simulink model "TxSteering_RxMVDR_4x4_HDL_IQ"  (R2021b)
settings: Solver=FixedStepDiscrete  StartTime=0.0  StopTime=stoptime  RelTol=1e-3
PreLoadFcn:
  | model_init
InitFcn:
  | model_init
model workspace (MAT data in the model file):
  socvcb = containers.Map
  socvcb.serialization.keys = {}
  socvcb.serialization.values = {}
  socvcb.serialization.uniformity = 0
  socvcb.serialization.keyType = 'double'
  socvcb.serialization.valueType = 'any'
values from neighbouring files (symbols this model uses):
  fc = ConverterSampleRate/4    (= 491520000)    [model_init.m]
  FPGAClkRate = DataSampleRate/VectorSamplingFactor    (= 245760000)    [model_init.m]
  movavg_bitshift = nextpow2(sqrt(windowSize))    [model_init.m]
  mvdrPipelineDelay = covMatDelay+movAvgDelay+matrixDivDelay+normResponseDelay    [model_init.m]
  NCO_bits = 14    [model_init.m]
  numArrayElements = 4    [model_init.m]
  S2MM_frame_size = testSrc1.FrameLength*testSrc1.SamplesPerSymbol*3    [model_init.m]
  testSrc1 = struct()    [model_init.m]
  testSrc2 = struct()    [model_init.m]
  windowSize = 4096    [model_init.m]
undefined symbols (not defined in the file or in its folder): j, physconst
libraries: hdlsllib x19, simulink x12, dspsrcs4 x2, embsystolicmatrixops x1, embreciprocals x1, dsphdlsigops x1, commrfcorlib x1
(part 1 of 3)
Description:
  | MVDR RFSoC example for ZCU111
  | 
  | Copyright 2021 The MathWorks, Inc.
settings Model: DataTypeOverride=Off  Creator=mfornero  LastModifiedBy=tmealey
settings SolverCC: AlgebraicLoopSolver=TrustRegion
settings DataIOCC: SaveOutput=off  SaveTime=off  ReturnWorkspaceOutputs=off
settings OptimizationCC: BlockReduction=off  ConditionallyExecuteInputs=off  DefaultParameterBehavior=Inlined  LifeSpan=inf
settings DebuggingCC: AlgebraicLoopMsg=error  SingleTaskRateTransMsg=error  ParameterPrecisionLossMsg=none  PregeneratedLibrarySubsystemCodeDiagnostic=none  StrictBusMsg=ErrorOnBusTreatedAsVector  SFUnexpectedBacktrackingDiag=warning  SFNoUnconditionalDefaultTransitionDiag=warning  SFExecutionAtInitializationDiag=none  SFMachineParentedDataDiag=warning  ArithmeticOperatorsInVariantConditions=warning
settings HardwareCC: ProdBitPerPointer=32  ProdBitPerSizeT=32  ProdBitPerPtrDiffT=32  ProdLargestAtomicFloat=None  ProdIntDivRoundTo=Undefined  ProdEndianess=Unspecified  ProdWordSize=32  ProdHWDeviceType=ASIC/FPGA->ASIC/FPGA  ProdEqTarget=off
settings SFSimCC: SimUseLocalCustomCode=off  CustomCodeUndefinedFunction=UseInterfaceOnly
settings RTWCC: RTWUseLocalCustomCode=off
settings CodeAppCC: StateflowObjectComments=on
settings GRTTargetCC: TargetLangStandard=C89/C90 (ANSI)
settings ConfigComp: CovMetricSettings=dw  CovSaveCumulativeToWorkspaceVar=on  CovSaveSingleToWorkspaceVar=on  CovExternalEMLEnable=off

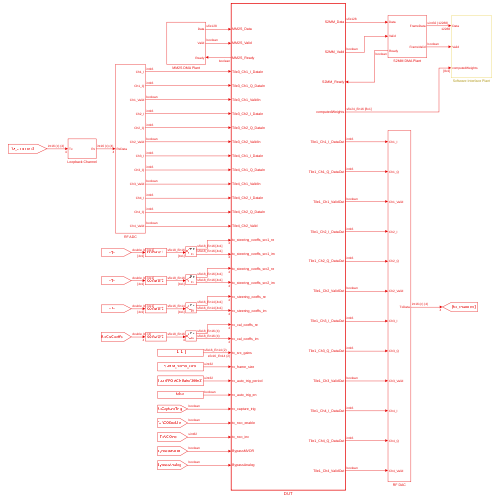
[thumbnail: Simulink's stored preview of the top-level diagram]
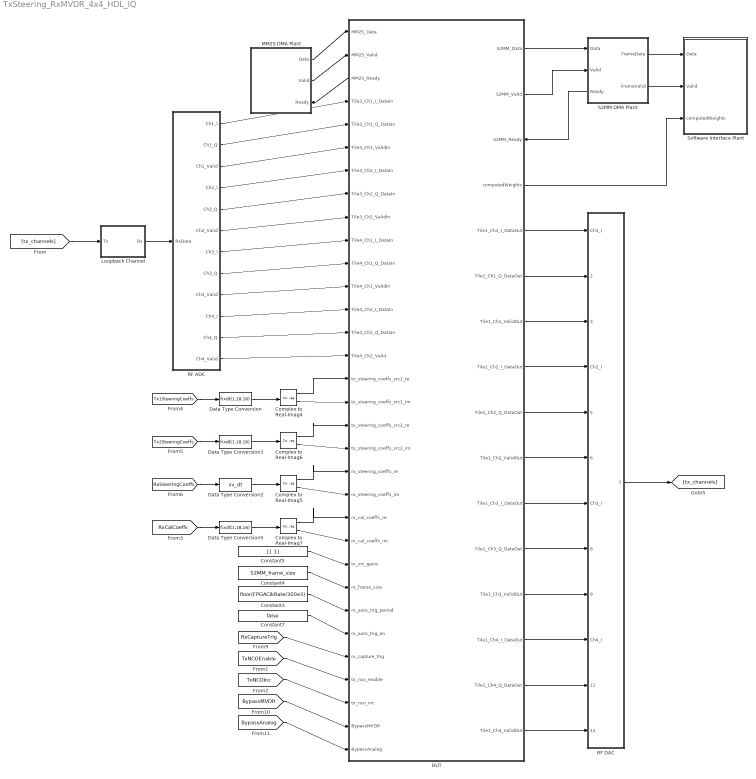
== system TxSteering_RxMVDR_4x4_HDL_IQ ==
  Complex to Real-Imag{4..7} (4 alike) : ComplexToRealImag
  Constant3 : Constant  Value=floor(FPGAClkRate/300e3)  OutDataTypeStr=uint32  SampleTime=-1
  Constant4 : Constant  Value=S2MM_frame_size  OutDataTypeStr=uint32  SampleTime=-1
  Constant5 : Constant  Value=[1 1]  OutDataTypeStr=tx_gain_dt  SampleTime=-1
  Constant7 : Constant  Value=false  SampleTime=-1
  DUT : Subsystem  TreatAsAtomicUnit=on
      settings: PortSchema="{\"entries\":[{\"content\":{\"sides\":[{\"content\":{\"connectorIds\":[\"In1\",\"In2\",\"Out16\",\"In3\",\"In4\",\"In5\",\"In6\",\"In7\",\"In8\",\"In9\",\"In10\",\"In11\",\"In12\",\"In13\",\"In14\",\"In15\",\"In16\",\"In17\",\"In18\",\"In19\",\"In20\",\"In21\",\"In22\",\"In23\",\"In24\",\"In25\",\"In26\",\"In27\",\"In28\",\"In29\",\"In30\",\"In31\"]},\"type\":\"ConnectorPlacement.EquallySpacedRectSide\",\"uuid\":\"5cbbc5c1-13a2-4dd5-b798-0d6aa5a3512c\"},{\"content\":{\"connectorIds\":[\"Out1\",\"Out2\",\"In32\",\"Out3\",\"Out4\",\"Out5\",\"Out6\",\"Out7\",\"Out8\",\"Out9\",\"Out10\",\"Out11\",\"Out12\",\"Out13\",\"Out14\",\"Out15\"],\"side\":\"RIGHT\"},\"type\":\"ConnectorPlacement.EquallySpacedRectSide\",\"uuid\":\"078c6bc6-159b-4e6a-9020-aaf50b1c87f6\"},{\"content\":{\"connectorIds\":[],\"side\":\"TOP\"},\"type\":\"ConnectorPlacement.EquallySpacedRectSide\",\"uuid\":\"5dec20bf-c028-4555-acb0-00d4e0bd1eb1\"},{\"content\":{\"connectorIds\":[],\"side\":\"HIDDEN\"},\"type\":\"ConnectorPlacement.EquallySpacedRectSide\",\"uuid\":\"f104c99f-3c00-46d1-a3ab-da9a095ae20c\"}]},\"type\":\"ConnectorPlacement.EquallySpacedConnector\",\"uuid\":\"99ff154b-6e8c-428f-8f67-53aff3cd9053\"}],\"packageUris\":[\"http://schema.mathworks.com/mf0/Connector/R2020b\"],\"version\":\"1.0\"}"
  Data Type Conversion : DataTypeConversion  OutDataTypeStr=fixdt(1,18,16)
  Data Type Conversion2 : DataTypeConversion  OutDataTypeStr=sv_dt
  Data Type Conversion3 : DataTypeConversion  OutDataTypeStr=fixdt(1,18,16)
  Data Type Conversion5 : DataTypeConversion  OutDataTypeStr=fixdt(1,18,16)
  Loopback Channel : Subsystem
  MM2S DMA Plant : Subsystem
      settings: PortSchema="{\"entries\":[{\"content\":{\"sides\":[{\"content\":{\"connectorIds\":[]},\"type\":\"ConnectorPlacement.EquallySpacedRectSide\",\"uuid\":\"6e5a1ec8-43bd-4e5c-bb67-adc7e52f765e\"},{\"content\":{\"connectorIds\":[\"Out1\",\"Out2\",\"In1\"],\"side\":\"RIGHT\"},\"type\":\"ConnectorPlacement.EquallySpacedRectSide\",\"uuid\":\"3e14b147-97a5-457d-828e-9dc648279d0e\"},{\"content\":{\"connectorIds\":[],\"side\":\"TOP\"},\"type\":\"ConnectorPlacement.EquallySpacedRectSide\",\"uuid\":\"b499ca48-b31e-4779-aede-04dca658d330\"},{\"content\":{\"connectorIds\":[],\"side\":\"HIDDEN\"},\"type\":\"ConnectorPlacement.EquallySpacedRectSide\",\"uuid\":\"e46e2562-9ab1-42db-980c-487b803af873\"}]},\"type\":\"ConnectorPlacement.EquallySpacedConnector\",\"uuid\":\"234057b8-4ead-4b5a-9893-76ff1204f271\"}],\"packageUris\":[\"http://schema.mathworks.com/mf0/Connector/R2020b\"],\"version\":\"1.0\"}"
  RF ADC : Subsystem
  RF DAC : Subsystem
  S2MM DMA Plant : Subsystem
      settings: PortSchema="{\"entries\":[{\"content\":{\"sides\":[{\"content\":{\"connectorIds\":[\"In1\",\"In2\",\"Out3\"]},\"type\":\"ConnectorPlacement.EquallySpacedRectSide\",\"uuid\":\"f5aebce5-d24c-432e-8d9d-6ae810fc0a64\"},{\"content\":{\"connectorIds\":[\"Out1\",\"Out2\"],\"side\":\"RIGHT\"},\"type\":\"ConnectorPlacement.EquallySpacedRectSide\",\"uuid\":\"87d7b61c-1b18-489c-87d0-263bc891b967\"},{\"content\":{\"connectorIds\":[],\"side\":\"TOP\"},\"type\":\"ConnectorPlacement.EquallySpacedRectSide\",\"uuid\":\"c0471b66-642d-47c1-93a8-85d0262e809a\"},{\"content\":{\"connectorIds\":[],\"side\":\"HIDDEN\"},\"type\":\"ConnectorPlacement.EquallySpacedRectSide\",\"uuid\":\"468d2625-6b9b-4b39-93eb-7f122a4e72a5\"}]},\"type\":\"ConnectorPlacement.EquallySpacedConnector\",\"uuid\":\"6af60fba-ab37-47d2-9d8a-dd48226214e6\"}],\"packageUris\":[\"http://schema.mathworks.com/mf0/Connector/R2020b\"],\"version\":\"1.0\"}"
  Software Interface Plant : Subsystem
  wires:
  Complex to Real-Imag4/2 -> DUT/16(tx_steering_coeffs_src1_im)
  [BypassAnalog] -> DUT/31(BypassAnalog)
  Complex to Real-Imag5/2 -> DUT/20(rx_steering_coeffs_im)
  Complex to Real-Imag6/2 -> DUT/18(tx_steering_coeffs_src2_im)
  Complex to Real-Imag6/1 -> DUT/17(tx_steering_coeffs_src2_re)
  Complex to Real-Imag5/1 -> DUT/19(rx_steering_coeffs_re)
  Data Type Conversion3/1 -> Complex to Real-Imag6/1
  Complex to Real-Imag4/1 -> DUT/15(tx_steering_coeffs_src1_re)
  Data Type Conversion2/1 -> Complex to Real-Imag5/1
  [Tx1SteeringCoeffs] -> Data Type Conversion/1
  Data Type Conversion/1 -> Complex to Real-Imag4/1
  Constant5/1 -> DUT/23(tx_src_gains)
  Constant7/1 -> DUT/26(rx_auto_trig_en)
  Constant3/1 -> DUT/25(rx_auto_trig_period)
  Constant4/1 -> DUT/24(rx_frame_size)
  [RxCaptureTrig] -> DUT/27(rx_capture_trig)
  Data Type Conversion5/1 -> Complex to Real-Imag7/1
  Complex to Real-Imag7/1 -> DUT/21(rx_cal_coeffs_re)
  Complex to Real-Imag7/2 -> DUT/22(rx_cal_coeffs_im)
  [RxCalCoeffs] -> Data Type Conversion5/1
  DUT/16(MM2S_Ready) -> MM2S DMA Plant/1(Ready)
  MM2S DMA Plant/2(Valid) -> DUT/2(MM2S_Valid)
  MM2S DMA Plant/1(Data) -> DUT/1(MM2S_Data)
  [BypassMVDR] -> DUT/30(BypassMVDR)
  DUT/4(Tile1_Ch1_I_DataOut) -> RF DAC/1(Ch1_I)
  DUT/5(Tile1_Ch1_Q_DataOut) -> RF DAC/2(Ch1_Q)
  DUT/6(Tile1_Ch1_ValidOut) -> RF DAC/3(Ch1_Valid)
  DUT/7(Tile1_Ch2_I_DataOut) -> RF DAC/4(Ch2_I)
  DUT/8(Tile1_Ch2_Q_DataOut) -> RF DAC/5(Ch2_Q)
  DUT/9(Tile1_Ch2_ValidOut) -> RF DAC/6(Ch2_Valid)
  DUT/10(Tile1_Ch3_I_DataOut) -> RF DAC/7(Ch3_I)
  DUT/11(Tile1_Ch3_Q_DataOut) -> RF DAC/8(Ch3_Q)
  DUT/12(Tile1_Ch3_ValidOut) -> RF DAC/9(Ch3_Valid)
  DUT/13(Tile1_Ch4_I_DataOut) -> RF DAC/10(Ch4_I)
  DUT/14(Tile1_Ch4_Q_DataOut) -> RF DAC/11(Ch4_Q)
  DUT/15(Tile1_Ch4_ValidOut) -> RF DAC/12(Ch4_Valid)
  RF DAC/1(TxData) -> [tx_channels]
  RF ADC/1(Ch1_I) -> DUT/3("Tile3_Ch1_I_DataIn ")
  RF ADC/2(Ch1_Q) -> DUT/4(Tile3_Ch1_Q_DataIn)
  RF ADC/4(Ch2_I) -> DUT/6(Tile3_Ch2_I_DataIn)
  RF ADC/5(Ch2_Q) -> DUT/7(Tile3_Ch2_Q_DataIn)
  RF ADC/7(Ch3_I) -> DUT/9(Tile4_Ch1_I_DataIn)
  RF ADC/8(Ch3_Q) -> DUT/10(Tile4_Ch1_Q_DataIn)
  RF ADC/10(Ch4_I) -> DUT/12(Tile4_Ch2_I_DataIn)
  RF ADC/11(Ch4_Q) -> DUT/13(Tile4_Ch2_Q_DataIn)
  RF ADC/3(Ch1_Valid) -> DUT/5(Tile3_Ch1_ValidIn)
  RF ADC/6(Ch2_Valid) -> DUT/8(Tile3_Ch2_ValidIn)
  RF ADC/9(Ch3_Valid) -> DUT/11(Tile4_Ch1_ValidIn)
  RF ADC/12(Ch4_Valid) -> DUT/14(Tile4_Ch2_Valid)
  [tx_channels] -> Loopback Channel/1(Tx)
  Loopback Channel/1(Rx) -> RF ADC/1(RxData)
  [TxNCOEnable] -> DUT/28(tx_nco_enable)
  [TxNCOInc] -> DUT/29(tx_nco_inc)
  S2MM DMA Plant/3(Ready) -> DUT/32(S2MM_Ready)
  DUT/2(S2MM_Valid) -> S2MM DMA Plant/2(Valid)
  DUT/1(S2MM_Data) -> S2MM DMA Plant/1(Data)
  S2MM DMA Plant/1(FrameData) -> Software Interface Plant/1(Data)
  S2MM DMA Plant/2(FrameValid) -> Software Interface Plant/2(Valid)
  DUT/3(computedWeights) -> Software Interface Plant/3(computedWeights)
  [Tx2SteeringCoeffs] -> Data Type Conversion3/1
  [RxSteeringCoeffs] -> Data Type Conversion2/1

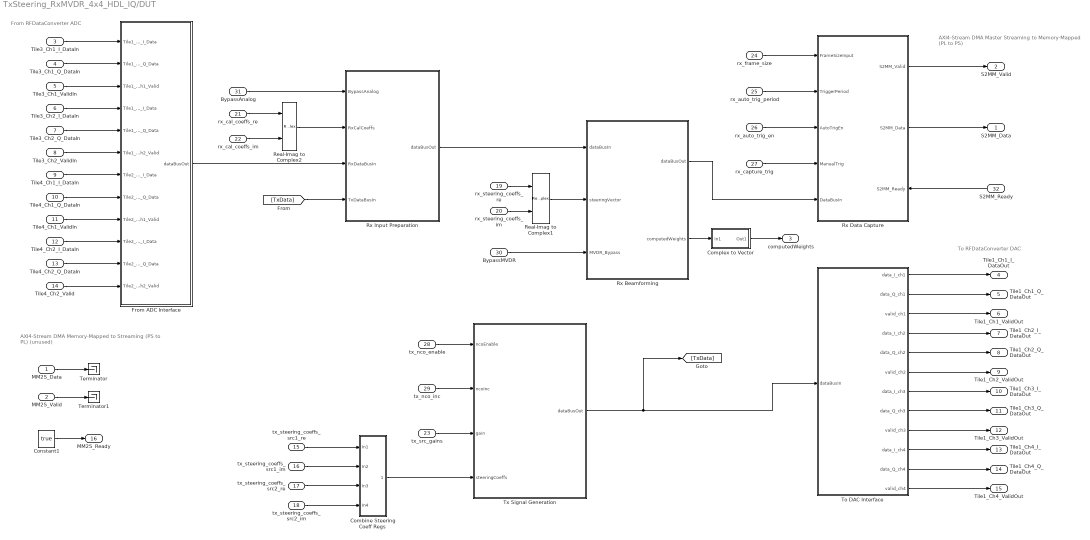
== system TxSteering_RxMVDR_4x4_HDL_IQ/DUT ==
  note: AXI4-Stream DMA Master
      | Streaming to Memory-Mapped (PL to PS)
  note: AXI4-Stream DMA
      | Memory-Mapped to Streaming (PS to PL)
      | (unused)
  note: From RFDataConverter ADC
  note: To RFDataConverter DAC
  MM2S_Data : Inport
  MM2S_Valid : Inport  Port=2
  "Tile3_Ch1_I_DataIn " : Inport  Port=3
  Tile3_Ch1_Q_DataIn : Inport  Port=4
  Tile3_Ch1_ValidIn : Inport  Port=5
  Tile3_Ch2_I_DataIn : Inport  Port=6
  Tile3_Ch2_Q_DataIn : Inport  Port=7
  Tile3_Ch2_ValidIn : Inport  Port=8
  Tile4_Ch1_I_DataIn : Inport  Port=9
  Tile4_Ch1_Q_DataIn : Inport  Port=10
  Tile4_Ch1_ValidIn : Inport  Port=11
  Tile4_Ch2_I_DataIn : Inport  Port=12
  Tile4_Ch2_Q_DataIn : Inport  Port=13
  Tile4_Ch2_Valid : Inport  Port=14
  tx_steering_coeffs_src1_re : Inport  Port=15  PortDimensions=NumChan
  tx_steering_coeffs_src1_im : Inport  Port=16  PortDimensions=NumChan
  tx_steering_coeffs_src2_re : Inport  Port=17  PortDimensions=NumChan
  tx_steering_coeffs_src2_im : Inport  Port=18  PortDimensions=NumChan
  rx_steering_coeffs_re : Inport  Port=19  PortDimensions=NumChan
  rx_steering_coeffs_im : Inport  Port=20  PortDimensions=NumChan
  rx_cal_coeffs_re : Inport  Port=21  PortDimensions=NumChan
  rx_cal_coeffs_im : Inport  Port=22  PortDimensions=NumChan
  tx_src_gains : Inport  Port=23  OutDataTypeStr=tx_gain_dt
  rx_frame_size : Inport  Port=24
  rx_auto_trig_period : Inport  Port=25
  rx_auto_trig_en : Inport  Port=26
  rx_capture_trig : Inport  Port=27
  tx_nco_enable : Inport  Port=28
  tx_nco_inc : Inport  Port=29
  BypassMVDR : Inport  Port=30
  BypassAnalog : Inport  Port=31
  S2MM_Ready : Inport  Port=32
  Combine Steering Coeff Regs : Subsystem
  Complex to Vector : Subsystem
  Constant1 : Constant  Value=true  OutDataTypeStr=boolean  SampleTime=-1
  From ADC Interface : Subsystem
  Real-Imag to Complex1 : RealImagToComplex
  Real-Imag to Complex2 : RealImagToComplex
  Rx Beamforming : Subsystem
  Rx Data Capture : Subsystem
      settings: PortSchema="{\"entries\":[{\"content\":{\"sides\":[{\"content\":{\"connectorIds\":[\"In1\",\"In2\",\"In3\",\"In4\",\"In5\"]},\"type\":\"ConnectorPlacement.EquallySpacedRectSide\",\"uuid\":\"3ce440ad-60a3-40a1-9abc-8b07e8479e74\"},{\"content\":{\"connectorIds\":[\"Out1\",\"Out2\",\"In6\"],\"side\":\"RIGHT\"},\"type\":\"ConnectorPlacement.EquallySpacedRectSide\",\"uuid\":\"92cb9a6e-31c8-4c68-811d-5cb9de201228\"},{\"content\":{\"connectorIds\":[],\"side\":\"TOP\"},\"type\":\"ConnectorPlacement.EquallySpacedRectSide\",\"uuid\":\"4ff664a1-3d68-43c3-89c1-825c045b6984\"},{\"content\":{\"connectorIds\":[],\"side\":\"HIDDEN\"},\"type\":\"ConnectorPlacement.EquallySpacedRectSide\",\"uuid\":\"ea40c324-81e0-4145-89f3-1e0de81d6070\"}]},\"type\":\"ConnectorPlacement.EquallySpacedConnector\",\"uuid\":\"89aac716-5ee7-4b56-a06e-6874cb9890cb\"}],\"packageUris\":[\"http://schema.mathworks.com/mf0/Connector/R2020b\"],\"version\":\"1.0\"}"
  Rx Input Preparation : Subsystem
  Terminator : Terminator
  Terminator1 : Terminator
  To DAC Interface : Subsystem
  Tx Signal Generation : Subsystem
  S2MM_Data : Outport  VectorParamsAs1DForOutWhenUnconnected=off
  S2MM_Valid : Outport  Port=2  VectorParamsAs1DForOutWhenUnconnected=off
  computedWeights : Outport  Port=3
  Tile1_Ch1_I_DataOut : Outport  Port=4  VectorParamsAs1DForOutWhenUnconnected=off
  Tile1_Ch1_Q_DataOut : Outport  Port=5  VectorParamsAs1DForOutWhenUnconnected=off
  Tile1_Ch1_ValidOut : Outport  Port=6  VectorParamsAs1DForOutWhenUnconnected=off
  Tile1_Ch2_I_DataOut : Outport  Port=7  VectorParamsAs1DForOutWhenUnconnected=off
  Tile1_Ch2_Q_DataOut : Outport  Port=8  VectorParamsAs1DForOutWhenUnconnected=off
  Tile1_Ch2_ValidOut : Outport  Port=9  VectorParamsAs1DForOutWhenUnconnected=off
  Tile1_Ch3_I_DataOut : Outport  Port=10  VectorParamsAs1DForOutWhenUnconnected=off
  Tile1_Ch3_Q_DataOut : Outport  Port=11  VectorParamsAs1DForOutWhenUnconnected=off
  Tile1_Ch3_ValidOut : Outport  Port=12  VectorParamsAs1DForOutWhenUnconnected=off
  Tile1_Ch4_I_DataOut : Outport  Port=13  VectorParamsAs1DForOutWhenUnconnected=off
  Tile1_Ch4_Q_DataOut : Outport  Port=14  VectorParamsAs1DForOutWhenUnconnected=off
  Tile1_Ch4_ValidOut : Outport  Port=15  VectorParamsAs1DForOutWhenUnconnected=off
  MM2S_Ready : Outport  Port=16  VectorParamsAs1DForOutWhenUnconnected=off
  wires:
  Constant1/1 -> MM2S_Ready/1
  S2MM_Ready/1 -> Rx Data Capture/6(S2MM_Ready)
  rx_frame_size/1 -> Rx Data Capture/1(FrameSizeInput)
  rx_auto_trig_period/1 -> Rx Data Capture/2(TriggerPeriod)
  rx_auto_trig_en/1 -> Rx Data Capture/3(AutoTrigEn)
  rx_capture_trig/1 -> Rx Data Capture/4(ManualTrig)
  Rx Data Capture/1(S2MM_Valid) -> S2MM_Valid/1
  Rx Data Capture/2(S2MM_Data) -> S2MM_Data/1
  "Tile3_Ch1_I_DataIn "/1 -> From ADC Interface/1("Tile1_Ch1_I_Data ")
  Tile3_Ch1_ValidIn/1 -> From ADC Interface/3(Tile1_Ch1_Valid)
  Tile3_Ch1_Q_DataIn/1 -> From ADC Interface/2(Tile1_Ch1_Q_Data)
  Tile3_Ch2_I_DataIn/1 -> From ADC Interface/4(Tile1_Ch2_I_Data)
  Tile3_Ch2_ValidIn/1 -> From ADC Interface/6(Tile1_Ch2_Valid)
  Tile3_Ch2_Q_DataIn/1 -> From ADC Interface/5(Tile1_Ch2_Q_Data)
  Tile4_Ch1_I_DataIn/1 -> From ADC Interface/7(Tile2_Ch1_I_Data)
  Tile4_Ch1_ValidIn/1 -> From ADC Interface/9(Tile2_Ch1_Valid)
  Tile4_Ch1_Q_DataIn/1 -> From ADC Interface/8(Tile2_Ch1_Q_Data)
  Tile4_Ch2_I_DataIn/1 -> From ADC Interface/10(Tile2_Ch2_I_Data)
  Tile4_Ch2_Valid/1 -> From ADC Interface/12(Tile2_Ch2_Valid)
  Tile4_Ch2_Q_DataIn/1 -> From ADC Interface/11(Tile2_Ch2_Q_Data)
  MM2S_Data/1 -> Terminator/1
  MM2S_Valid/1 -> Terminator1/1
  To DAC Interface/1(data_I_ch1) -> Tile1_Ch1_I_DataOut/1
  To DAC Interface/2(data_Q_ch1) -> Tile1_Ch1_Q_DataOut/1
  To DAC Interface/3(valid_ch1) -> Tile1_Ch1_ValidOut/1
  To DAC Interface/4(data_I_ch2) -> Tile1_Ch2_I_DataOut/1
  To DAC Interface/5(data_Q_ch2) -> Tile1_Ch2_Q_DataOut/1
  To DAC Interface/6(valid_ch2) -> Tile1_Ch2_ValidOut/1
  To DAC Interface/7(data_I_ch3) -> Tile1_Ch3_I_DataOut/1
  To DAC Interface/8(data_Q_ch3) -> Tile1_Ch3_Q_DataOut/1
  To DAC Interface/9(valid_ch3) -> Tile1_Ch3_ValidOut/1
  To DAC Interface/10(data_I_ch4) -> Tile1_Ch4_I_DataOut/1
  To DAC Interface/11(data_Q_ch4) -> Tile1_Ch4_Q_DataOut/1
  To DAC Interface/12(valid_ch4) -> Tile1_Ch4_ValidOut/1
  rx_steering_coeffs_im/1 -> Real-Imag to Complex1/2
  Real-Imag to Complex1/1 -> Rx Beamforming/2(steeringVector)
  rx_steering_coeffs_re/1 -> Real-Imag to Complex1/1
  tx_steering_coeffs_src1_re/1 -> Combine Steering Coeff Regs/1(In1)
  tx_steering_coeffs_src1_im/1 -> Combine Steering Coeff Regs/2(In2)
  tx_steering_coeffs_src2_re/1 -> Combine Steering Coeff Regs/3(In3)
  tx_steering_coeffs_src2_im/1 -> Combine Steering Coeff Regs/4(In4)
  Rx Beamforming/1(dataBusOut) -> Rx Data Capture/5(DataBusIn)
  [TxData] -> Rx Input Preparation/4(TxDataBusIn)
  BypassMVDR/1 -> Rx Beamforming/3(MVDR_Bypass)
  BypassAnalog/1 -> Rx Input Preparation/1(BypassAnalog)
  rx_cal_coeffs_re/1 -> Real-Imag to Complex2/1
  rx_cal_coeffs_im/1 -> Real-Imag to Complex2/2
  Real-Imag to Complex2/1 -> Rx Input Preparation/2(RxCalCoeffs)
  Tx Signal Generation/1(dataBusOut) -> [TxData], To DAC Interface/1(dataBusIn)
  Combine Steering Coeff Regs/1(steeringCoeffs) -> Tx Signal Generation/4(steeringCoeffs)
  tx_src_gains/1 -> Tx Signal Generation/3(gain)
  Rx Input Preparation/1(dataBusOut) -> Rx Beamforming/1(dataBusIn)
  From ADC Interface/1(dataBusOut) -> Rx Input Preparation/3(RxDataBusIn)
  tx_nco_inc/1 -> Tx Signal Generation/2(ncoInc)
  tx_nco_enable/1 -> Tx Signal Generation/1(ncoEnable)
  Rx Beamforming/2(computedWeights) -> Complex to Vector/1(In1)
  Complex to Vector/1(Out1) -> computedWeights/1

== system TxSteering_RxMVDR_4x4_HDL_IQ/Loopback Channel ==
  Tx : Inport
  Apply Channel Noise : Subsystem
  Apply Phase/Amplitude imbalance : Subsystem
  Data Type Conversion : DataTypeConversion  OutDataTypeStr=fixdt(1,16,14)  ConvertRealWorld=Stored Integer (SI)
  Data Type Conversion1 : DataTypeConversion  OutDataTypeStr=double
  Data Type Conversion2 : DataTypeConversion  OutDataTypeStr=fixdt(1,16,14)
  Data Type Conversion3 : DataTypeConversion  OutDataTypeStr=int16  ConvertRealWorld=Stored Integer (SI)
  Delay1 : Delay  DelayLength=1
  Rx : Outport
  wires:
  Tx/1 -> Delay1/1
  Delay1/1 -> Data Type Conversion/1
  Data Type Conversion/1 -> Data Type Conversion1/1
  Data Type Conversion2/1 -> Data Type Conversion3/1
  Data Type Conversion3/1 -> Rx/1
  Apply Channel Noise/1(Out1) -> Data Type Conversion2/1
  Data Type Conversion1/1 -> Apply Phase/Amplitude imbalance/1(In1)
  Apply Phase/Amplitude imbalance/1(Out1) -> Apply Channel Noise/1(In1)

== system TxSteering_RxMVDR_4x4_HDL_IQ/MM2S DMA Plant ==
  Ready : Inport
  Constant6 : Constant  Value=false  SampleTime=-1
  Constant7 : Constant  Value=0  OutDataTypeStr=fixdt(0,128,0)  SampleTime=-1
  Terminator : Terminator
  Data : Outport
  Valid : Outport  Port=2
  wires:
  Constant7/1 -> Data/1
  Constant6/1 -> Valid/1
  Ready/1 -> Terminator/1

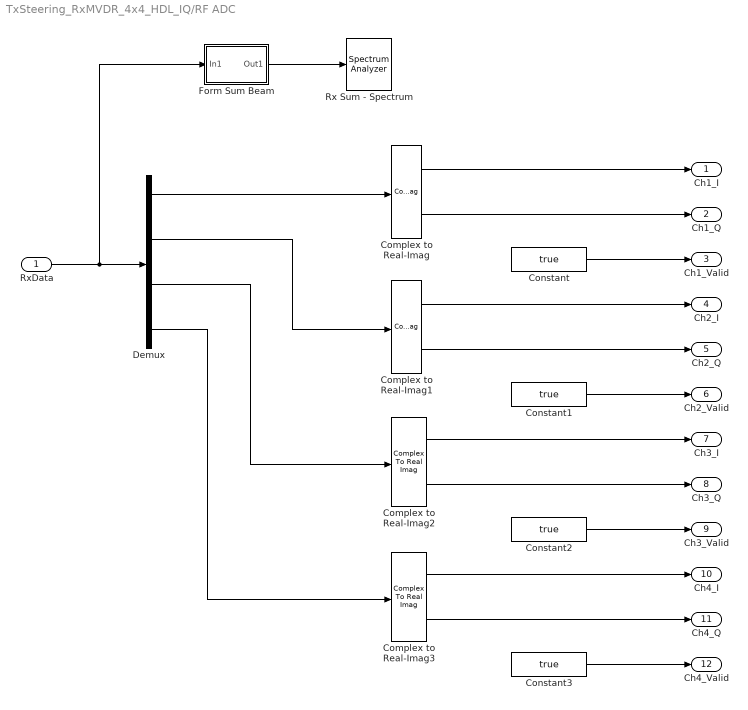
== system TxSteering_RxMVDR_4x4_HDL_IQ/RF ADC ==
  RxData : Inport
  Complex to Real-Imag{,1..3} (4 alike) : ComplexToRealImag
  Constant{,1..3} (4 alike) : Constant  Value=true  SampleTime=-1
  Demux : Demux
  Form Sum Beam : Subsystem
  Rx Sum - Spectrum : SpectrumAnalyzer
  Ch1_I : Outport
  Ch1_Q : Outport  Port=2
  Ch1_Valid : Outport  Port=3
  Ch2_I : Outport  Port=4
  Ch2_Q : Outport  Port=5
  Ch2_Valid : Outport  Port=6
  Ch3_I : Outport  Port=7
  Ch3_Q : Outport  Port=8
  Ch3_Valid : Outport  Port=9
  Ch4_I : Outport  Port=10
  Ch4_Q : Outport  Port=11
  Ch4_Valid : Outport  Port=12
  wires:
  Demux/4 -> Complex to Real-Imag3/1
  Complex to Real-Imag1/1 -> Ch2_I/1
  Demux/2 -> Complex to Real-Imag1/1
  Complex to Real-Imag2/2 -> Ch3_Q/1
  Complex to Real-Imag3/1 -> Ch4_I/1
  Demux/3 -> Complex to Real-Imag2/1
  Complex to Real-Imag2/1 -> Ch3_I/1
  Complex to Real-Imag3/2 -> Ch4_Q/1
  Complex to Real-Imag/2 -> Ch1_Q/1
  Complex to Real-Imag/1 -> Ch1_I/1
  Complex to Real-Imag1/2 -> Ch2_Q/1
  Constant/1 -> Ch1_Valid/1
  Demux/1 -> Complex to Real-Imag/1
  Constant1/1 -> Ch2_Valid/1
  Constant2/1 -> Ch3_Valid/1
  Constant3/1 -> Ch4_Valid/1
  RxData/1 -> Form Sum Beam/1(In1), Demux/1
  Form Sum Beam/1(Out1) -> Rx Sum - Spectrum/1

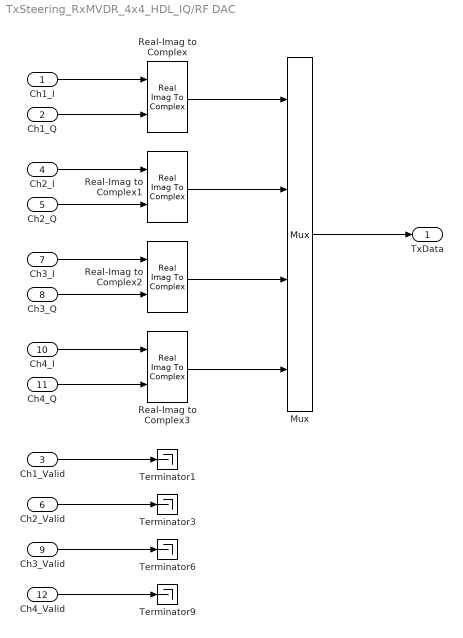
== system TxSteering_RxMVDR_4x4_HDL_IQ/RF DAC ==
  Ch1_I : Inport
  Ch1_Q : Inport  Port=2
  Ch1_Valid : Inport  Port=3
  Ch2_I : Inport  Port=4
  Ch2_Q : Inport  Port=5
  Ch2_Valid : Inport  Port=6
  Ch3_I : Inport  Port=7
  Ch3_Q : Inport  Port=8
  Ch3_Valid : Inport  Port=9
  Ch4_I : Inport  Port=10
  Ch4_Q : Inport  Port=11
  Ch4_Valid : Inport  Port=12
  Mux : Mux
  Real-Imag to Complex{,1..3} (4 alike) : RealImagToComplex
  Terminator{1,3,6,9} (4 alike) : Terminator
  TxData : Outport
  wires:
  Ch2_Q/1 -> Real-Imag to Complex1/2
  Ch2_Valid/1 -> Terminator3/1
  Ch3_Valid/1 -> Terminator6/1
  Ch1_Valid/1 -> Terminator1/1
  Ch4_I/1 -> Real-Imag to Complex3/1
  Ch4_Q/1 -> Real-Imag to Complex3/2
  Ch3_Q/1 -> Real-Imag to Complex2/2
  Ch4_Valid/1 -> Terminator9/1
  Ch1_Q/1 -> Real-Imag to Complex/2
  Ch1_I/1 -> Real-Imag to Complex/1
  Ch2_I/1 -> Real-Imag to Complex1/1
  Ch3_I/1 -> Real-Imag to Complex2/1
  Real-Imag to Complex/1 -> Mux/1
  Real-Imag to Complex1/1 -> Mux/2
  Real-Imag to Complex2/1 -> Mux/3
  Real-Imag to Complex3/1 -> Mux/4
  Mux/1 -> TxData/1

== system TxSteering_RxMVDR_4x4_HDL_IQ/S2MM DMA Plant ==
  Data : Inport
  Valid : Inport  Port=2
  AXI Stream Deserializer : MATLAB Function  TreatAsAtomicUnit=on  mask{FRAME_SIZE=S2MM_frame_size}
      mask prompts: FRAME_SIZE "Frame size:"
  Constant10 : Constant  Value=true  SampleTime=-1
  Delay : Delay  DelayLength=1
  Delay1 : Delay  DelayLength=1
  Unpack to uint32 : Subsystem
  FrameData : Outport
  FrameValid : Outport  Port=2
  Ready : Outport  Port=3
  wires:
  Data/1 -> AXI Stream Deserializer/1(data_i)
  Valid/1 -> AXI Stream Deserializer/2(valid_i)
  Constant10/1 -> Ready/1
  AXI Stream Deserializer/1(data_o) -> Delay/1
  AXI Stream Deserializer/2(valid_o) -> Delay1/1
  Unpack to uint32/1(dataOut) -> FrameData/1
  Unpack to uint32/2(validOut) -> FrameValid/1
  Delay/1 -> Unpack to uint32/1(dataIn)
  Delay1/1 -> Unpack to uint32/2(validIn)

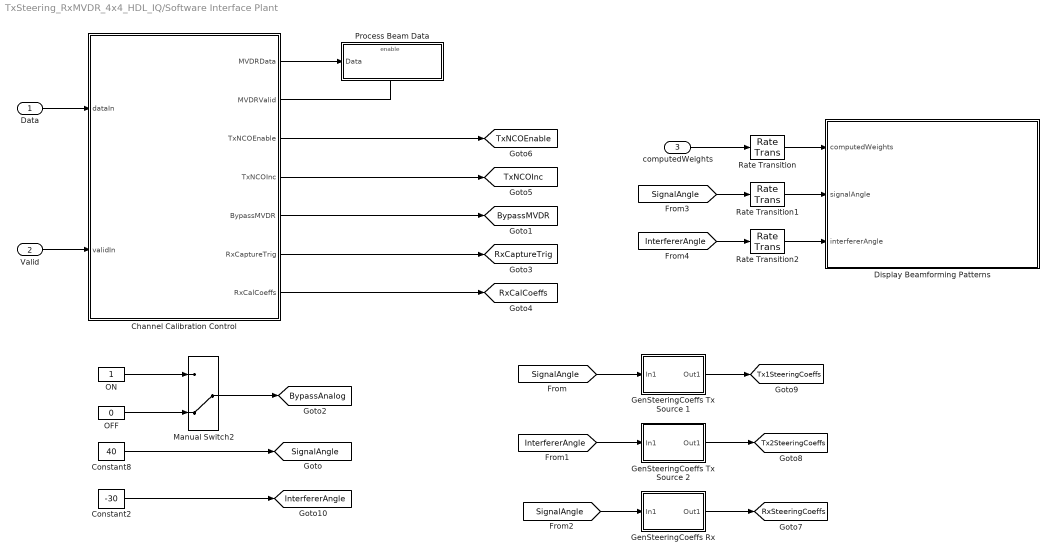
== system TxSteering_RxMVDR_4x4_HDL_IQ/Software Interface Plant ==
  Data : Inport
  Valid : Inport  Port=2
  computedWeights : Inport  Port=3
  Channel Calibration Control : MATLAB Function  TreatAsAtomicUnit=on
  Constant2 : Constant  Value=-30  OutDataTypeStr=double  SampleTime=-1
  Constant8 : Constant  Value=40  OutDataTypeStr=double  SampleTime=-1
  Display Beamforming Patterns : MATLAB Function  TreatAsAtomicUnit=on
  GenSteeringCoeffs Rx : Subsystem
  GenSteeringCoeffs Tx Source 1 : Subsystem
  GenSteeringCoeffs Tx Source 2 : Subsystem
  Manual Switch2 : ManualSwitch  CurrentSetting=0
  OFF : Constant  Value=0  OutDataTypeStr=boolean  SampleTime=-1
  ON : Constant  OutDataTypeStr=boolean  SampleTime=-1
  Process Beam Data : Subsystem
  Rate Transition : RateTransition  OutPortSampleTimeOpt=Multiple of input port sample time  OutPortSampleTimeMultiple=256
  Rate Transition1 : RateTransition  OutPortSampleTimeOpt=Multiple of input port sample time  OutPortSampleTimeMultiple=256
  Rate Transition2 : RateTransition  OutPortSampleTimeOpt=Multiple of input port sample time  OutPortSampleTimeMultiple=256
  tag scope: BypassAnalog=global, BypassMVDR=global, InterfererAngle=global, RxCalCoeffs=global, RxCaptureTrig=global, RxSteeringCoeffs=global, SignalAngle=global, Tx1SteeringCoeffs=global, Tx2SteeringCoeffs=global, TxNCOEnable=global, TxNCOInc=global
  wires:
  Channel Calibration Control/5(BypassMVDR) -> [BypassMVDR]
  OFF/1 -> Manual Switch2/2
  Manual Switch2/1 -> [BypassAnalog]
  ON/1 -> Manual Switch2/1
  Data/1 -> Channel Calibration Control/1(dataIn)
  Valid/1 -> Channel Calibration Control/2(validIn)
  Channel Calibration Control/6(RxCaptureTrig) -> [RxCaptureTrig]
  Channel Calibration Control/4(TxNCOInc) -> [TxNCOInc]
  Channel Calibration Control/3(TxNCOEnable) -> [TxNCOEnable]
  Channel Calibration Control/7(RxCalCoeffs) -> [RxCalCoeffs]
  Channel Calibration Control/1(MVDRData) -> Process Beam Data/1(Data)
  GenSteeringCoeffs Rx/1(Out1) -> [RxSteeringCoeffs]
  GenSteeringCoeffs Tx Source 2/1(Out1) -> [Tx2SteeringCoeffs]
  GenSteeringCoeffs Tx Source 1/1(Out1) -> [Tx1SteeringCoeffs]
  Constant8/1 -> [SignalAngle]
  Constant2/1 -> [InterfererAngle]
  [SignalAngle] -> GenSteeringCoeffs Tx Source 1/1(In1)
  [InterfererAngle] -> GenSteeringCoeffs Tx Source 2/1(In1)
  [SignalAngle] -> GenSteeringCoeffs Rx/1(In1)
  computedWeights/1 -> Rate Transition/1
  [SignalAngle] -> Rate Transition1/1
  [InterfererAngle] -> Rate Transition2/1
  Rate Transition/1 -> Display Beamforming Patterns/1(computedWeights)
  Rate Transition1/1 -> Display Beamforming Patterns/2(signalAngle)
  Rate Transition2/1 -> Display Beamforming Patterns/3(interfererAngle)
  Channel Calibration Control/2(MVDRValid) -> Process Beam Data/Enable

== system TxSteering_RxMVDR_4x4_HDL_IQ/DUT/Combine Steering Coeff Regs ==
  In1 : Inport
  In2 : Inport  Port=2
  In3 : Inport  Port=3
  In4 : Inport  Port=4
  Real-Imag to Complex : RealImagToComplex
  Real-Imag to Complex2 : RealImagToComplex
  Vector Concatenate : Concatenate
  steeringCoeffs : Outport
  wires:
  In1/1 -> Real-Imag to Complex/1
  In2/1 -> Real-Imag to Complex/2
  In4/1 -> Real-Imag to Complex2/2
  In3/1 -> Real-Imag to Complex2/1
  Real-Imag to Complex/1 -> Vector Concatenate/1
  Real-Imag to Complex2/1 -> Vector Concatenate/2
  Vector Concatenate/1 -> steeringCoeffs/1

== system TxSteering_RxMVDR_4x4_HDL_IQ/DUT/Complex to Vector ==
  In1 : Inport
  Complex to Real-Imag : ComplexToRealImag
  Matrix Concatenate : Concatenate  Mode=Multidimensional array
  Out1 : Outport
  wires:
  In1/1 -> Complex to Real-Imag/1
  Complex to Real-Imag/1 -> Matrix Concatenate/1
  Complex to Real-Imag/2 -> Matrix Concatenate/2
  Matrix Concatenate/1 -> Out1/1

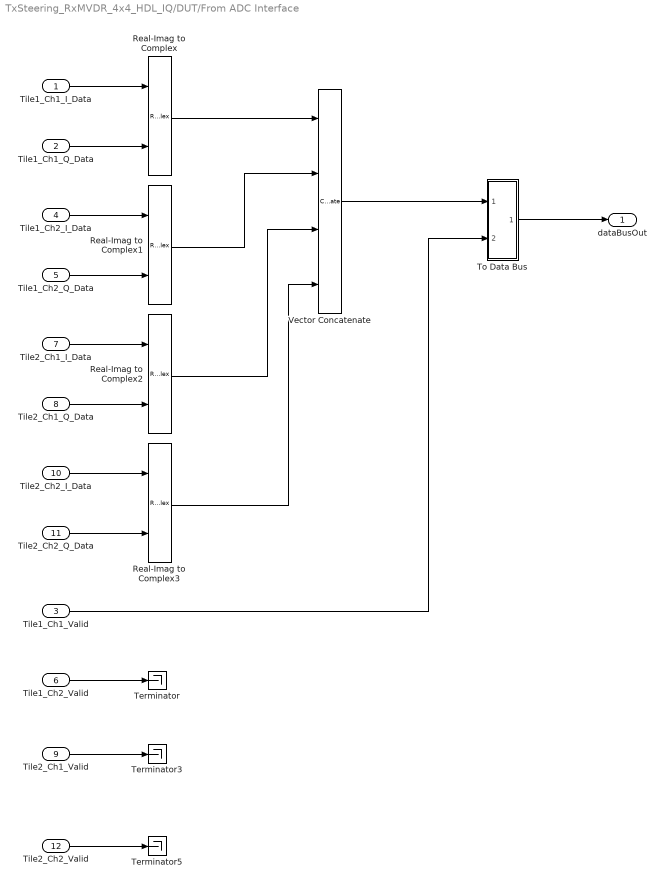
== system TxSteering_RxMVDR_4x4_HDL_IQ/DUT/From ADC Interface ==
  "Tile1_Ch1_I_Data " : Inport
  Tile1_Ch1_Q_Data : Inport  Port=2
  Tile1_Ch1_Valid : Inport  Port=3
  Tile1_Ch2_I_Data : Inport  Port=4
  Tile1_Ch2_Q_Data : Inport  Port=5
  Tile1_Ch2_Valid : Inport  Port=6
  Tile2_Ch1_I_Data : Inport  Port=7
  Tile2_Ch1_Q_Data : Inport  Port=8
  Tile2_Ch1_Valid : Inport  Port=9
  Tile2_Ch2_I_Data : Inport  Port=10
  Tile2_Ch2_Q_Data : Inport  Port=11
  Tile2_Ch2_Valid : Inport  Port=12
  Real-Imag to Complex{,1..3} (4 alike) : RealImagToComplex
  Terminator : Terminator
  Terminator3 : Terminator
  Terminator5 : Terminator
  To Data Bus : Subsystem  mask(To Data Bus){dummy=0}
      mask help: Create a streaming Data Bus from Data and Valid signals.
      mask Display:
      | port_label('input',1,'data');
      | port_label('input',2,'valid');
  Vector Concatenate : Concatenate  NumInputs=4  Mode=Multidimensional array  ConcatenateDimension=2
  dataBusOut : Outport  VectorParamsAs1DForOutWhenUnconnected=off
  wires:
  Tile1_Ch2_Valid/1 -> Terminator/1
  Tile2_Ch1_Valid/1 -> Terminator3/1
  Tile2_Ch2_Valid/1 -> Terminator5/1
  Real-Imag to Complex/1 -> Vector Concatenate/1
  Real-Imag to Complex1/1 -> Vector Concatenate/2
  Real-Imag to Complex2/1 -> Vector Concatenate/3
  Real-Imag to Complex3/1 -> Vector Concatenate/4
  "Tile1_Ch1_I_Data "/1 -> Real-Imag to Complex/1
  Tile1_Ch1_Q_Data/1 -> Real-Imag to Complex/2
  Tile1_Ch2_I_Data/1 -> Real-Imag to Complex1/1
  Tile1_Ch2_Q_Data/1 -> Real-Imag to Complex1/2
  Tile2_Ch1_I_Data/1 -> Real-Imag to Complex2/1
  Tile2_Ch1_Q_Data/1 -> Real-Imag to Complex2/2
  Tile2_Ch2_I_Data/1 -> Real-Imag to Complex3/1
  Tile2_Ch2_Q_Data/1 -> Real-Imag to Complex3/2
  Vector Concatenate/1 -> To Data Bus/1(data)
  Tile1_Ch1_Valid/1 -> To Data Bus/2(valid)
  To Data Bus/1(bus) -> dataBusOut/1

== system TxSteering_RxMVDR_4x4_HDL_IQ/DUT/Rx Beamforming ==
  dataBusIn : Inport
  steeringVector : Inport  Port=2
  MVDR_Bypass : Inport  Port=3
  Input Gate : Subsystem
  MVDR : Subsystem
  Output Selector : Subsystem
  dataBusOut : Outport
  computedWeights : Outport  Port=2
  wires:
  Output Selector/1(DataOut) -> dataBusOut/1
  MVDR_Bypass/1 -> Output Selector/1(BypassEn), Input Gate/1(BypassEn)
  steeringVector/1 -> MVDR/2(steeringVector)
  MVDR/1(DataBusOut) -> Output Selector/3(MVDR_Input)
  dataBusIn/1 -> Input Gate/2(dataBusIn)
  Input Gate/2(MVDRDataBus) -> MVDR/1(dataBusIn)
  Input Gate/1(BypassDataBus) -> Output Selector/2(Bypass_Input)
  MVDR/2(computedWeights) -> computedWeights/1

== system TxSteering_RxMVDR_4x4_HDL_IQ/DUT/Rx Data Capture ==
  FrameSizeInput : Inport
  TriggerPeriod : Inport  Port=2
  AutoTrigEn : Inport  Port=3
  ManualTrig : Inport  Port=4
  Bus Element In : Inport  Port=5  PortName=DataBusIn  Element=data
  Bus Element In1 : Inport  Port=5  PortName=DataBusIn  Element=valid
  S2MM_Ready : Inport  Port=6
  CaptureTriggerControl : Subsystem
  Delay{,1..5} (6 alike) : Delay  DelayLength=1
  FIFOControl : Subsystem
      settings: PortSchema="{\"entries\":[{\"content\":{\"sides\":[{\"content\":{\"connectorIds\":[\"In1\",\"In2\",\"In3\"]},\"type\":\"ConnectorPlacement.EquallySpacedRectSide\",\"uuid\":\"ccba886f-6d80-4f19-97b3-7ae55bfa6a76\"},{\"content\":{\"connectorIds\":[\"Out1\",\"In4\"],\"side\":\"RIGHT\"},\"type\":\"ConnectorPlacement.EquallySpacedRectSide\",\"uuid\":\"cf0e26ed-7a0e-4f19-ac3f-2da55ea62b3c\"},{\"content\":{\"connectorIds\":[],\"side\":\"TOP\"},\"type\":\"ConnectorPlacement.EquallySpacedRectSide\",\"uuid\":\"e4948715-49d6-4073-841d-7fe6792f6b27\"},{\"content\":{\"connectorIds\":[],\"side\":\"HIDDEN\"},\"type\":\"ConnectorPlacement.EquallySpacedRectSide\",\"uuid\":\"cea0585b-9d24-4f9e-a212-0bcf2233187e\"}]},\"type\":\"ConnectorPlacement.EquallySpacedConnector\",\"uuid\":\"c48b1748-38f6-42dc-ab34-329a94089643\"}],\"packageUris\":[\"http://schema.mathworks.com/mf0/Connector/R2020b\"],\"version\":\"1.0\"}"
  "Stream FIFO " : Subsystem
      settings: PortSchema="{\"entries\":[{\"content\":{\"sides\":[{\"content\":{\"connectorIds\":[\"In1\",\"In2\",\"Out3\"]},\"type\":\"ConnectorPlacement.EquallySpacedRectSide\",\"uuid\":\"f5aebce5-d24c-432e-8d9d-6ae810fc0a64\"},{\"content\":{\"connectorIds\":[\"Out1\",\"Out2\",\"In3\"],\"side\":\"RIGHT\"},\"type\":\"ConnectorPlacement.EquallySpacedRectSide\",\"uuid\":\"87d7b61c-1b18-489c-87d0-263bc891b967\"},{\"content\":{\"connectorIds\":[],\"side\":\"TOP\"},\"type\":\"ConnectorPlacement.EquallySpacedRectSide\",\"uuid\":\"c0471b66-642d-47c1-93a8-85d0262e809a\"},{\"content\":{\"connectorIds\":[],\"side\":\"HIDDEN\"},\"type\":\"ConnectorPlacement.EquallySpacedRectSide\",\"uuid\":\"468d2625-6b9b-4b39-93eb-7f122a4e72a5\"}]},\"type\":\"ConnectorPlacement.EquallySpacedConnector\",\"uuid\":\"6af60fba-ab37-47d2-9d8a-dd48226214e6\"}],\"packageUris\":[\"http://schema.mathworks.com/mf0/Connector/R2020b\"],\"version\":\"1.0\"}"
  S2MM_Valid : Outport  VectorParamsAs1DForOutWhenUnconnected=off
  S2MM_Data : Outport  Port=2  VectorParamsAs1DForOutWhenUnconnected=off
  wires:
  FrameSizeInput/1 -> Delay2/1
  S2MM_Ready/1 -> "Stream FIFO "/3(readyIn)
  "Stream FIFO "/2(ValidOut) -> S2MM_Valid/1
  FIFOControl/1(validOut) -> "Stream FIFO "/2(validIn)
  "Stream FIFO "/3(readyOut) -> FIFOControl/4(fifoReady)
  Delay2/1 -> FIFOControl/2(FrameSize)
  "Stream FIFO "/1(dataOut) -> S2MM_Data/1
  Bus Element In1/1 -> Delay1/1
  Delay/1 -> "Stream FIFO "/1(dataIn)
  Bus Element In/1 -> Delay/1
  Delay1/1 -> FIFOControl/1(validIn)
  CaptureTriggerControl/1(Trig) -> FIFOControl/3(Trigger)
  Delay3/1 -> CaptureTriggerControl/1(AutoTrigPeriod)
  TriggerPeriod/1 -> Delay3/1
  Delay5/1 -> CaptureTriggerControl/2(AutoTrigEn)
  Delay4/1 -> CaptureTriggerControl/3(ManualTrig)
  AutoTrigEn/1 -> Delay5/1
  ManualTrig/1 -> Delay4/1

== system TxSteering_RxMVDR_4x4_HDL_IQ/DUT/Rx Input Preparation ==
  BypassAnalog : Inport
  RxCalCoeffs : Inport  Port=2
  RxDataBusIn : Inport  Port=3
  TxDataBusIn : Inport  Port=4
  Apply Calibration Coefficients : Subsystem
  Delay1 : Delay  DelayLength=1
  Delay2 : Delay  DelayLength=1
  From Data Bus : Subsystem  mask(From Data Bus){dummy=0}
      mask help: Convert a streaming Data Bus to individual Data and Valid signals.
      mask Display:
      | port_label('output',1,'data');
      | port_label('output',2,'valid');
  Switch : Switch  Criteria=u2 > Threshold
  To Data Bus : Subsystem  mask(To Data Bus){dummy=0}
      mask help: Create a streaming Data Bus from Data and Valid signals.
      mask Display:
      | port_label('input',1,'data');
      | port_label('input',2,'valid');
  dataBusOut : Outport  VectorParamsAs1DForOutWhenUnconnected=off
  wires:
  RxCalCoeffs/1 -> Apply Calibration Coefficients/3(coeffIn)
  Apply Calibration Coefficients/2(validOut) -> To Data Bus/2(valid)
  Apply Calibration Coefficients/1(dataOut) -> To Data Bus/1(data)
  From Data Bus/1(data) -> Apply Calibration Coefficients/1(dataIn)
  Delay2/1 -> Switch/3
  Delay1/1 -> dataBusOut/1
  BypassAnalog/1 -> Switch/2
  Switch/1 -> Delay1/1
  TxDataBusIn/1 -> Switch/1
  To Data Bus/1(bus) -> Delay2/1
  RxDataBusIn/1 -> From Data Bus/1(bus)
  From Data Bus/2(valid) -> Apply Calibration Coefficients/2(validIn)

== system TxSteering_RxMVDR_4x4_HDL_IQ/DUT/To DAC Interface ==
  dataBusIn : Inport
  Complex to Real-Imag : ComplexToRealImag
  Data Type Conversion : DataTypeConversion  OutDataTypeStr=int16  ConvertRealWorld=Stored Integer (SI)
  Demux : Demux
  Demux1 : Demux
  From Data Bus : Subsystem  mask(From Data Bus){dummy=0}
      mask help: Convert a streaming Data Bus to individual Data and Valid signals.
      mask Display:
      | port_label('output',1,'data');
      | port_label('output',2,'valid');
  data_I_ch1 : Outport
  data_Q_ch1 : Outport  Port=2
  valid_ch1 : Outport  Port=3
  data_I_ch2 : Outport  Port=4
  data_Q_ch2 : Outport  Port=5
  valid_ch2 : Outport  Port=6
  data_I_ch3 : Outport  Port=7
  data_Q_ch3 : Outport  Port=8
  valid_ch3 : Outport  Port=9
  data_I_ch4 : Outport  Port=10
  data_Q_ch4 : Outport  Port=11
  valid_ch4 : Outport  Port=12
  wires:
  dataBusIn/1 -> From Data Bus/1(bus)
  From Data Bus/1(data) -> Data Type Conversion/1
  Demux/1 -> data_I_ch1/1
  Demux1/1 -> data_Q_ch1/1
  From Data Bus/2(valid) -> valid_ch1/1, valid_ch2/1, valid_ch4/1, valid_ch3/1
  Demux/2 -> data_I_ch2/1
  Demux1/2 -> data_Q_ch2/1
  Demux/3 -> data_I_ch3/1
  Demux1/3 -> data_Q_ch3/1
  Demux/4 -> data_I_ch4/1
  Demux1/4 -> data_Q_ch4/1
  Data Type Conversion/1 -> Complex to Real-Imag/1
  Complex to Real-Imag/1 -> Demux/1
  Complex to Real-Imag/2 -> Demux1/1

== system TxSteering_RxMVDR_4x4_HDL_IQ/DUT/Tx Signal Generation ==
  ncoEnable : Inport
  ncoInc : Inport  Port=2
  gain : Inport  Port=3
  steeringCoeffs : Inport  Port=4
  Calibration NCO : Subsystem
  Combine Channels : Subsystem
  Demux : Demux  Outputs=2
  Generate Steering Channels : Subsystem  TreatAsAtomicUnit=on
  Multiport Switch : MultiPortSwitch  DataPortOrder=Zero-based contiguous  Inputs=2  zeroidx=on
  To Data Bus : Subsystem  mask(To Data Bus){dummy=0}
      mask help: Create a streaming Data Bus from Data and Valid signals.
      mask Display:
      | port_label('input',1,'data');
      | port_label('input',2,'valid');
  To Data Bus1 : Subsystem  mask(To Data Bus){dummy=0}
      mask help: Create a streaming Data Bus from Data and Valid signals.
      mask Display:
      | port_label('input',1,'data');
      | port_label('input',2,'valid');
  Tx Source LUT : Subsystem
  Tx Sources - Spectrum : SpectrumAnalyzer  NumInputPorts=2
  dataBusOut : Outport
  wires:
  gain/1 -> Generate Steering Channels/3(gain)
  steeringCoeffs/1 -> Generate Steering Channels/4(steeringCoeffs)
  Generate Steering Channels/1(dataOut) -> Combine Channels/1(dataIn)
  Generate Steering Channels/2(validOut) -> Combine Channels/2(validIn)
  Tx Source LUT/1(dataOut) -> Demux/1, Generate Steering Channels/1(dataIn)
  Tx Source LUT/2(validOut) -> Generate Steering Channels/2(validIn)
  Combine Channels/2(validOut) -> To Data Bus/2(valid)
  Combine Channels/1(dataOut) -> To Data Bus/1(data)
  Demux/1 -> Tx Sources - Spectrum/1  "Tx Source 1"
  Demux/2 -> Tx Sources - Spectrum/2  "Tx Source 2"
  ncoInc/1 -> Calibration NCO/1(inc)
  Calibration NCO/1(dataOut) -> To Data Bus1/1(data)
  Calibration NCO/2(validOut) -> To Data Bus1/2(valid)
  ncoEnable/1 -> Multiport Switch/1
  To Data Bus1/1(bus) -> Multiport Switch/3
  To Data Bus/1(bus) -> Multiport Switch/2
  Multiport Switch/1 -> dataBusOut/1

== system TxSteering_RxMVDR_4x4_HDL_IQ/Loopback Channel/Apply Channel Noise ==
  In1 : Inport
  Add : Sum
  Colored Noise : dspsrcs4/Colored Noise  Color=white  InverseFrequencyPower=1  BoundedOutput=off  NumChannels=4  OutputDataType=double  SamplesPerFrame=1  SampleTime=1/FPGAClkRate  RandomStream=mt19937ar with seed  Seed=67  SimulateUsing=Interpreted execution
      settings: SourceProductBaseCode=DS
  Colored Noise1 : dspsrcs4/Colored Noise  Color=white  InverseFrequencyPower=1  BoundedOutput=off  NumChannels=4  OutputDataType=double  SamplesPerFrame=1  SampleTime=1/FPGAClkRate  RandomStream=mt19937ar with seed  Seed=69  SimulateUsing=Interpreted execution
      settings: SourceProductBaseCode=DS
  Gain : Gain  Gain=3e-2
  Real-Imag to Complex : RealImagToComplex
  Reshape : Reshape
  Out1 : Outport
  wires:
  Colored Noise/1 -> Real-Imag to Complex/1
  Gain/1 -> Add/2
  Reshape/1 -> Gain/1
  Colored Noise1/1 -> Real-Imag to Complex/2
  In1/1 -> Add/1
  Real-Imag to Complex/1 -> Reshape/1
  Add/1 -> Out1/1

== system TxSteering_RxMVDR_4x4_HDL_IQ/Loopback Channel/Apply Phase//Amplitude imbalance ==
  In1 : Inport
  Constant : Constant  Value=[1.021*exp(-j*pi/12) 0.967*exp(j*pi/16) 0.945*exp(-j*pi/18) 1.072*exp(j*pi/11) ]  SampleTime=-1
  Gain : Gain  Gain=0.46
  Product : Product
  Out1 : Outport
  wires:
  Constant/1 -> Product/2
  In1/1 -> Gain/1
  Product/1 -> Out1/1
  Gain/1 -> Product/1

== system TxSteering_RxMVDR_4x4_HDL_IQ/RF ADC/Form Sum Beam ==
  In1 : Inport
  Data Type Conversion : DataTypeConversion  OutDataTypeStr=double
  Gain : Gain  Gain=1/(2^15)
  Sum of Elements : Sum  Inputs=+
  Out1 : Outport
  wires:
  Data Type Conversion/1 -> Gain/1
  In1/1 -> Data Type Conversion/1
  Sum of Elements/1 -> Out1/1
  Gain/1 -> Sum of Elements/1

== system TxSteering_RxMVDR_4x4_HDL_IQ/S2MM DMA Plant/Unpack to uint32 ==
  dataIn : Inport
  validIn : Inport  Port=2
  Enabled Subsystem : Subsystem  TreatAsAtomicUnit=on
  dataOut : Outport
  validOut : Outport  Port=2
  wires:
  Enabled Subsystem/1(dataOut) -> dataOut/1
  dataIn/1 -> Enabled Subsystem/1(dataIn)
  validIn/1 -> Enabled Subsystem/Enable, validOut/1

== system TxSteering_RxMVDR_4x4_HDL_IQ/Software Interface Plant/GenSteeringCoeffs Rx ==
  In1 : Inport
  Constant : Constant  Value=fc  SampleTime=-1
  Constant9 : Constant  Value=0  OutDataTypeStr=double  SampleTime=-1
  MATLAB System1 : MATLABSystem  System=phased.SteeringVector  PropagationSpeed=physconst( 'LightSpeed' )  IncludeElementResponse=off  NumPhaseShifterBits=0  EnablePolarization=off  SimulateUsing=Interpreted execution  SensorArray=sensorArray
      mask Type: phased.SteeringVector
      mask Display:
      | disp(['Steering' char(10) 'Vector']);
      | port_label('input',1,'Freq');
      | port_label('input',2,'Ang');
  Vector Concatenate : Concatenate  Mode=Multidimensional array
  Out1 : Outport
  wires:
  Vector Concatenate/1 -> MATLAB System1/2
  Constant/1 -> MATLAB System1/1
  In1/1 -> Vector Concatenate/1
  Constant9/1 -> Vector Concatenate/2
  MATLAB System1/1 -> Out1/1

== system TxSteering_RxMVDR_4x4_HDL_IQ/Software Interface Plant/GenSteeringCoeffs Tx Source 1 ==
  In1 : Inport
  Constant : Constant  Value=fc  SampleTime=-1
  Constant9 : Constant  Value=0  OutDataTypeStr=double  SampleTime=-1
  MATLAB System1 : MATLABSystem  System=phased.SteeringVector  PropagationSpeed=physconst( 'LightSpeed' )  IncludeElementResponse=off  NumPhaseShifterBits=0  EnablePolarization=off  SimulateUsing=Interpreted execution  SensorArray=sensorArray
      mask Type: phased.SteeringVector
      mask Display:
      | disp(['Steering' char(10) 'Vector']);
      | port_label('input',1,'Freq');
      | port_label('input',2,'Ang');
  Vector Concatenate : Concatenate  Mode=Multidimensional array
  Out1 : Outport
  wires:
  MATLAB System1/1 -> Out1/1
  Constant9/1 -> Vector Concatenate/2
  In1/1 -> Vector Concatenate/1
  Constant/1 -> MATLAB System1/1
  Vector Concatenate/1 -> MATLAB System1/2

== system TxSteering_RxMVDR_4x4_HDL_IQ/Software Interface Plant/GenSteeringCoeffs Tx Source 2 ==
  In1 : Inport
  Constant : Constant  Value=fc  SampleTime=-1
  Constant9 : Constant  Value=0  OutDataTypeStr=double  SampleTime=-1
  MATLAB System1 : MATLABSystem  System=phased.SteeringVector  PropagationSpeed=physconst( 'LightSpeed' )  IncludeElementResponse=off  NumPhaseShifterBits=0  EnablePolarization=off  SimulateUsing=Interpreted execution  SensorArray=sensorArray
      mask Type: phased.SteeringVector
      mask Display:
      | disp(['Steering' char(10) 'Vector']);
      | port_label('input',1,'Freq');
      | port_label('input',2,'Ang');
  Vector Concatenate : Concatenate  Mode=Multidimensional array
  Out1 : Outport
  wires:
  Vector Concatenate/1 -> MATLAB System1/2
  Constant/1 -> MATLAB System1/1
  In1/1 -> Vector Concatenate/1
  Constant9/1 -> Vector Concatenate/2
  MATLAB System1/1 -> Out1/1

== system TxSteering_RxMVDR_4x4_HDL_IQ/Software Interface Plant/Process Beam Data ==
  Data : Inport
  Enable : EnablePort
  AGC : commrfcorlib/AGC  LegacyMode=off  DetectorMethod=Rectifier  LoopMethod=Linear  UpdatePeriod=100  StepSize=0.1  AdaptationStepSize=1e-3  DesiredOutputPower=1  AveragingLength=256  MaximumGain=30  MaxPowerGain=60  GainOutputPort=off  InputPowerOutputPort=off  SimulateUsing=Interpreted execution
  QPSK Receiver : MATLAB Function  TreatAsAtomicUnit=on  mask{infoStruct=testSrc1}
      mask prompts: infoStruct "Source info struct:"
      mask init:
      | FrameLength = infoStruct.FrameLength;
      | SamplesPerSymbol = infoStruct.SamplesPerSymbol;
      | PreambleLength = infoStruct.PreambleLength;
      | mfCoeffs = infoStruct.mfCoeffs;
      | rrcCoeffs = infoStruct.rrcCoeffs;
  Reshape : Reshape  OutputDimensionality=Column vector (2-D)
  Rx Beam - Constellation : ConstellationDiagram
  To Workspace : ToWorkspace  VariableName=sim_beam_data  SampleTime=-1
      settings: Save2DSignal=2-D array (concatenate along first dimension)
  wires:
  Data/1 -> Reshape/1
  Reshape/1 -> QPSK Receiver/1(dataIn), To Workspace/1
  QPSK Receiver/1(dataOut) -> AGC/1
  AGC/1 -> Rx Beam - Constellation/1

== system TxSteering_RxMVDR_4x4_HDL_IQ/DUT/From ADC Interface/To Data Bus ==
  data : Inport
  valid : Inport  Port=2
  Bus Creator : BusCreator  Inputs=2
  bus : Outport  VectorParamsAs1DForOutWhenUnconnected=off
  wires:
  Bus Creator/1 -> bus/1
  data/1 -> Bus Creator/1  "data"
  valid/1 -> Bus Creator/2  "valid"

== system TxSteering_RxMVDR_4x4_HDL_IQ/DUT/Rx Beamforming/Input Gate ==
  BypassEn : Inport
  dataBusIn : Inport  Port=2
  AND : Logic  IconShape=distinctive  AllPortsSameDT=off  OutDataTypeStr=boolean
  From Data Bus : Subsystem  mask(From Data Bus){dummy=0}
      mask help: Convert a streaming Data Bus to individual Data and Valid signals.
      mask Display:
      | port_label('output',1,'data');
      | port_label('output',2,'valid');
  NOT : Logic  Operator=NOT  IconShape=distinctive  AllPortsSameDT=off  OutDataTypeStr=boolean
  To Data Bus : Subsystem  mask(To Data Bus){dummy=0}
      mask help: Create a streaming Data Bus from Data and Valid signals.
      mask Display:
      | port_label('input',1,'data');
      | port_label('input',2,'valid');
  To Data Bus1 : Subsystem  mask(To Data Bus){dummy=0}
      mask help: Create a streaming Data Bus from Data and Valid signals.
      mask Display:
      | port_label('input',1,'data');
      | port_label('input',2,'valid');
  BypassDataBus : Outport
  MVDRDataBus : Outport  Port=2
  wires:
  dataBusIn/1 -> From Data Bus/1(bus)
  To Data Bus/1(bus) -> BypassDataBus/1
  From Data Bus/1(data) -> To Data Bus1/1(data), To Data Bus/1(data)
  To Data Bus1/1(bus) -> MVDRDataBus/1
  From Data Bus/2(valid) -> To Data Bus/2(valid), AND/1
  BypassEn/1 -> NOT/1
  NOT/1 -> AND/2
  AND/1 -> To Data Bus1/2(valid)

== system TxSteering_RxMVDR_4x4_HDL_IQ/DUT/Rx Beamforming/MVDR ==
  dataBusIn : Inport
  steeringVector : Inport  Port=2
  Compute Weight Vector : Subsystem
  Form Beam : Subsystem
  Form Covariance Matrix : Subsystem
  Moving Average : Subsystem
  Normalize Response : Subsystem
  DataBusOut : Outport
  computedWeights : Outport  Port=2
  wires:
  dataBusIn/1 -> Form Covariance Matrix/1(dataBusIn), Form Beam/1(dataBusIn)
  Moving Average/1(dataOut) -> Compute Weight Vector/1(covarianceMatrix)
  Moving Average/2(validOut) -> Compute Weight Vector/2(validIn)
  steeringVector/1 -> Compute Weight Vector/3(steeringVector), Normalize Response/3(steeringVector)
  Compute Weight Vector/2(validOut) -> Normalize Response/2(validIn)
  Normalize Response/1(wOut) -> computedWeights/1, Form Beam/2(w)
  Compute Weight Vector/1(w) -> Normalize Response/1(wIn)
  Form Beam/1(dataBusOut) -> DataBusOut/1
  Form Covariance Matrix/1(dataOut) -> Moving Average/1(dataIn)
  Form Covariance Matrix/2(validOut) -> Moving Average/2(validIn)

== system TxSteering_RxMVDR_4x4_HDL_IQ/DUT/Rx Beamforming/Output Selector ==
  BypassEn : Inport
  Bypass_Input : Inport  Port=2
  MVDR_Input : Inport  Port=3
  Delay : Delay  DelayLength=1
  Delay1 : Delay  DelayLength=1
  Delay2 : Delay  DelayLength=1
  RepackageInput : Subsystem
  RepackageMVDR : Subsystem
  Switch : Switch  Criteria=u2 > Threshold
  DataOut : Outport
  wires:
  BypassEn/1 -> Delay2/1
  RepackageMVDR/1(Out1) -> Switch/3
  MVDR_Input/1 -> Delay1/1
  Bypass_Input/1 -> Delay/1
  RepackageInput/1(Out1) -> Switch/1
  Switch/1 -> DataOut/1
  Delay/1 -> RepackageInput/1(In1)
  Delay1/1 -> RepackageMVDR/1(In3)
  Delay2/1 -> Switch/2

== system TxSteering_RxMVDR_4x4_HDL_IQ/DUT/Rx Data Capture/CaptureTriggerControl ==
  AutoTrigPeriod : Inport
  AutoTrigEn : Inport  Port=2
  ManualTrig : Inport  Port=3
  AXI4-Lite Initial Value : Subsystem  mask(AXI4-Lite Initial Value){x0=uint32(floor(FPGAClkRate/2))}
      mask prompts: x0 "Initial value:"
      mask help: Set the initial value for an AXI4-Lite register.
      mask Display: fprintf('x0 = %g',x0);
  AutoTrigger : Subsystem
  Detect Increase : simulink/Logic and Bit Operations/Detect Increase  vinit=0.0  OutDataTypeStr=boolean
  Switch : Switch  Criteria=u2 > Threshold
  Trig : Outport
  wires:
  Switch/1 -> Detect Increase/1
  AutoTrigger/1(Trig) -> Switch/1
  AutoTrigEn/1 -> AutoTrigger/2(En), Switch/2
  ManualTrig/1 -> Switch/3
  AXI4-Lite Initial Value/1(Out1) -> AutoTrigger/1(MaxCount)
  AutoTrigPeriod/1 -> AXI4-Lite Initial Value/1(In1)
  Detect Increase/1 -> Trig/1

== system TxSteering_RxMVDR_4x4_HDL_IQ/DUT/Rx Data Capture/FIFOControl ==
  note: Pause counter when experiencing
      | backpressure from FIFO
  note: Handle edge-case if we're at the
      | max counter value and we have back-pressure, do not reset
      | just yet. Wait for back pressure to clear then a reset can be applied
  note: Count to N samples specified by AXI-lite consec frames input
  validIn : Inport
  FrameSize : Inport  Port=2
  Trigger : Inport  Port=3
  fifoReady : Inport  Port=4
  Data Type Conversion : DataTypeConversion  OutDataTypeStr=boolean
  HDL Counter : hdlsllib/Sources/HDL Counter  CountType=Free running  CountInit=0  CountStep=1  CountMax=25  CountFromType=Initial value  CountFrom=0  CountResetPort=on  CountLoadPort=off  CountEnbPort=on  CountDirPort=off  CountHitOutputPort=off  CountDataType=Unsigned  CountWordLen=32  CountFracLen=0  CountSampTime=1
  HandleDefaultValue : Subsystem
  Logical Operator : Logic  Inputs=3  IconShape=distinctive  AllPortsSameDT=off  OutDataTypeStr=boolean
  Logical Operator1 : Logic  IconShape=distinctive  AllPortsSameDT=off  OutDataTypeStr=boolean
  Logical Operator2 : Logic  IconShape=distinctive  AllPortsSameDT=off  OutDataTypeStr=boolean
  Relational Operator : RelationalOperator  Operator===  OutDataTypeStr=boolean  RndMeth=Simplest
  Signal Specification : SignalSpecification  OutDataTypeStr=boolean  Dimensions=1
  sr_latch : Subsystem
  validOut : Outport  VectorParamsAs1DForOutWhenUnconnected=off
  wires:
  Signal Specification/1 -> validOut/1  "DataCaptureEn"
  Trigger/1 -> sr_latch/1(S)
  sr_latch/1(Q) -> Logical Operator/1
  HDL Counter/1 -> Relational Operator/1, Data Type Conversion/1
  Logical Operator/1 -> HDL Counter/2  "En"
  Data Type Conversion/1 -> Logical Operator1/1
  Logical Operator1/1 -> Signal Specification/1
  Relational Operator/1 -> Logical Operator2/1, sr_latch/2(R)  "EndOfFrame"
  fifoReady/1 -> Logical Operator1/2, Logical Operator2/2, Logical Operator/2
  Logical Operator2/1 -> HDL Counter/1  "RstCount"
  FrameSize/1 -> HandleDefaultValue/1(In1)
  HandleDefaultValue/1(Out1) -> Relational Operator/2
  validIn/1 -> Logical Operator/3
